simulink model "Bio_fedbatch_PP2"  (R2022a)
settings: Solver=ode15s  StartTime=0.0  StopTime=tsim  RelTol=1e-4  AbsTol=1e-4
values from neighbouring files (symbols this model uses):
  Ts = 0.1    [BiofedBatchDT.m]    (also in Executable1.m; identification.m)
undefined symbols (not defined in the file or in its folder): in
libraries: sharedTrackingLibrary x1
settings Model: SimulationMode=accelerator  Creator=DELL  LastModifiedBy=LADES
settings SolverCC: SolverResetMethod=Robust
settings DataIOCC: ReturnWorkspaceOutputs=off

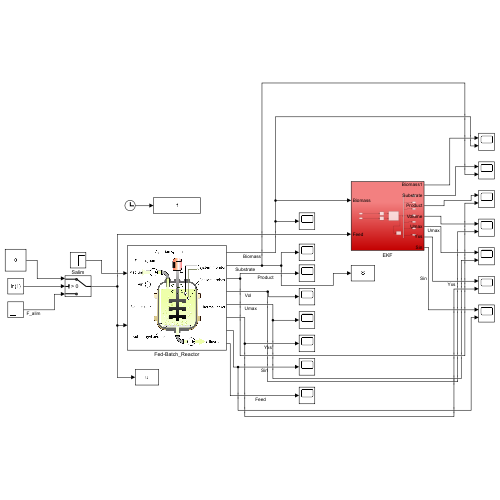
[thumbnail: Simulink's stored preview of the top-level diagram]
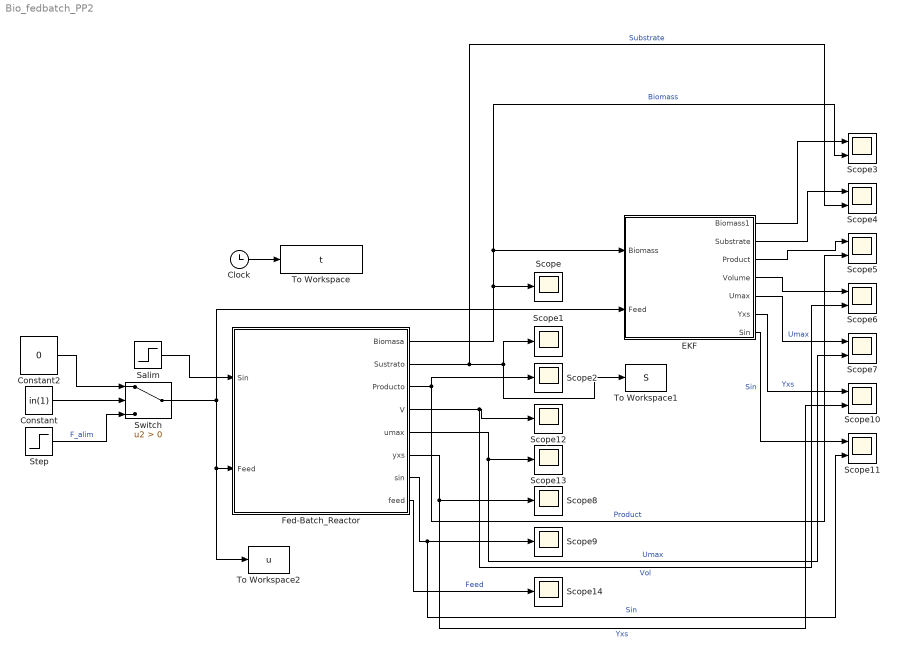
== system Bio_fedbatch_PP2 ==
  Clock : Clock
  Constant : Constant  Value=in(1)
  Constant2 : Constant  Value=0
  EKF : Subsystem
  Fed-Batch_Reactor : Subsystem
      mask Display: image('biorreactor.png'); % Use "Edit Image" on toolstrip to change.
  Salim : Step  Time=12  Before=10  After=10  SampleTime=0.1
  Scope{,1..2,8..9,12..14} (8 alike) : Scope
  Scope{3..7,10..11} (7 alike) : Scope  NumInputPorts=2
  Step : Step  Time=12  After=0.1  SampleTime=0
  Switch : Switch  Criteria=u2 > Threshold  SaturateOnIntegerOverflow=off  InputSameDT=off
  To Workspace : ToWorkspace  VariableName=t  SampleTime=0.1
  To Workspace1 : ToWorkspace  VariableName=S  SampleTime=0.1
  To Workspace2 : ToWorkspace  VariableName=u  SampleTime=0.1
  wires:
  Clock/1 -> To Workspace/1
  Fed-Batch_Reactor/2(Sustrato) -> Scope4/2, Scope1/1, To Workspace1/1  "Substrate"
  Fed-Batch_Reactor/1(Biomasa) -> EKF/1(Biomass), Scope3/2, Scope/1  "Biomass"
  Fed-Batch_Reactor/3(Producto) -> Scope2/1, Scope5/2  "Product"
  Fed-Batch_Reactor/6(yxs) -> Scope10/2, Scope8/1  "Yxs"
  Fed-Batch_Reactor/7(sin) -> Scope11/2, Scope9/1  "Sin"
  Fed-Batch_Reactor/4(V) -> Scope6/2, Scope12/1  "Vol"
  Fed-Batch_Reactor/5(umax) -> Scope7/2, Scope13/1  "Umax"
  Fed-Batch_Reactor/8(feed) -> Scope14/1  "Feed"
  Switch/1 -> To Workspace2/1, Fed-Batch_Reactor/2(Feed), EKF/2(Feed)
  EKF/1(Biomass1) -> Scope3/1
  EKF/2(Substrate) -> Scope4/1
  EKF/3(Product) -> Scope5/1
  EKF/4(Volume) -> Scope6/1
  EKF/5(Umax) -> Scope7/1  "Umax"
  EKF/6(Yxs) -> Scope10/1  "Yxs"
  EKF/7(Sin) -> Scope11/1  "Sin"
  Constant/1 -> Switch/2
  Constant2/1 -> Switch/1
  Step/1 -> Switch/3  "F_alim"
  Salim/1 -> Fed-Batch_Reactor/1(Sin)

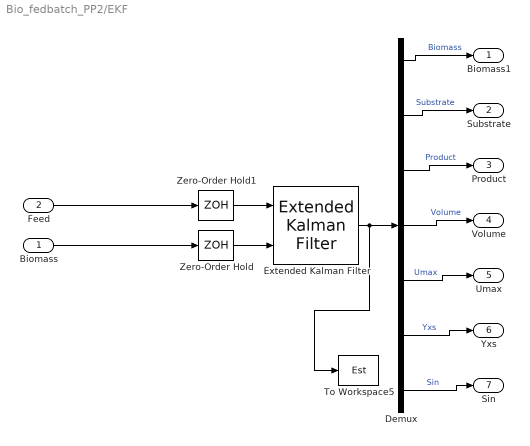
== system Bio_fedbatch_PP2/EKF ==
  Biomass : Inport
  Feed : Inport  Port=2
  Demux : Demux  Outputs=7
  Extended Kalman Filter : sharedTrackingLibrary/Extended Kalman Filter  StateTransitionFcn=BiofedBatchDT  HasStateTransitionJacobianFcn=off  HasAdditiveProcessNoise=Additive  ProcessNoise=[1e-3 1e-5 1e-3 1e-3 1e-1 1e-1 1e-1]  HasTimeVaryingProcessNoise=off  HasStateTransitionFcnExtraArgument=1  InitialState=x0  InitialStateCovariance=[1e-3 1e-5 1e-3 1e-3 1e-1 1e-1 1e-1]  MeasurementFcn1=FedBatchMeasFcn  HasMeasurementJacobianFcn1=off  HasMeasurementEnablePort1=off  HasAdditiveMeasurementNoise1=Additive  MeasurementNoise1=1e-3  HasTimeVaryingMeasurementNoise1=off  HasMeasurementFcnExtraArgument1=0  HasMeasurementWrapping1=off  MeasurementFcn2=myMeasurementFcn  HasMeasurementJacobianFcn2=off  HasMeasurementEnablePort2=off  HasAdditiveMeasurementNoise2=Additive  MeasurementNoise2=1  HasTimeVaryingMeasurementNoise2=off  HasMeasurementFcnExtraArgument2=0  HasMeasurementWrapping2=off  MeasurementFcn3=myMeasurementFcn  HasMeasurementJacobianFcn3=off  HasMeasurementEnablePort3=off  HasAdditiveMeasurementNoise3=Additive  MeasurementNoise3=1  HasTimeVaryingMeasurementNoise3=off  HasMeasurementFcnExtraArgument3=0  HasMeasurementWrapping3=off  MeasurementFcn4=myMeasurementFcn  HasMeasurementJacobianFcn4=off  HasMeasurementEnablePort4=off  HasAdditiveMeasurementNoise4=Additive  MeasurementNoise4=1  HasTimeVaryingMeasurementNoise4=off  HasMeasurementFcnExtraArgument4=0  HasMeasurementWrapping4=off  MeasurementFcn5=myMeasurementFcn  HasMeasurementJacobianFcn5=off  HasMeasurementEnablePort5=off  HasAdditiveMeasurementNoise5=Additive  MeasurementNoise5=1  HasTimeVaryingMeasurementNoise5=off  HasMeasurementFcnExtraArgument5=0  HasMeasurementWrapping5=off  EnableMultirate=off  StateTransitionFcnSampleTime=1  MeasurementFcn1SampleTime=1  MeasurementFcn2SampleTime=1  MeasurementFcn3SampleTime=1  MeasurementFcn4SampleTime=1  MeasurementFcn5SampleTime=1  UseCurrentEstimator=on  OutputStateCovariance=off  DataType=double  SampleTime=Ts  NumberOfMeasurements=1
      settings: SourceProductBaseCode=TF,AE,PW,CT,DR,ID,LP,NV,AR,RO,RR,UV,VE
  To Workspace5 : ToWorkspace  VariableName=Est  SampleTime=0.1
  Zero-Order Hold : ZeroOrderHold  SampleTime=Ts
  Zero-Order Hold1 : ZeroOrderHold  SampleTime=Ts
  Biomass1 : Outport
  Substrate : Outport  Port=2
  Product : Outport  Port=3
  Volume : Outport  Port=4
  Umax : Outport  Port=5
  Yxs : Outport  Port=6
  Sin : Outport  Port=7
  wires:
  Extended Kalman Filter/1 -> To Workspace5/1, Demux/1
  Demux/6 -> Yxs/1  "Yxs"
  Demux/2 -> Substrate/1  "Substrate"
  Feed/1 -> Zero-Order Hold1/1
  Zero-Order Hold/1 -> Extended Kalman Filter/2
  Zero-Order Hold1/1 -> Extended Kalman Filter/1
  Demux/1 -> Biomass1/1  "Biomass"
  Biomass/1 -> Zero-Order Hold/1
  Demux/4 -> Volume/1  "Volume"
  Demux/7 -> Sin/1  "Sin"
  Demux/3 -> Product/1  "Product"
  Demux/5 -> Umax/1  "Umax"

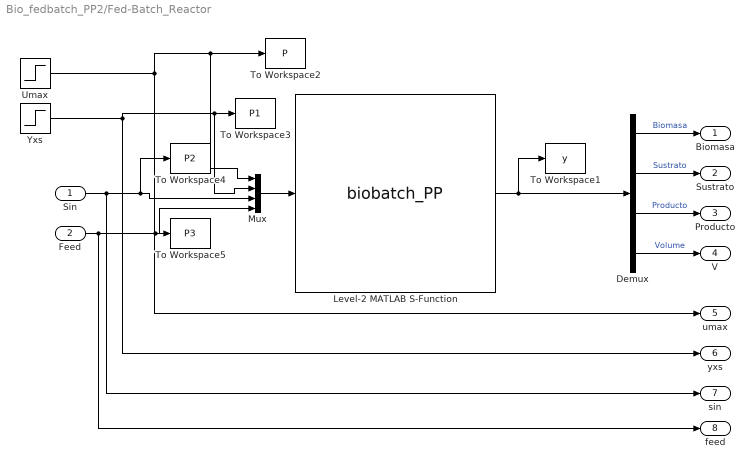
== system Bio_fedbatch_PP2/Fed-Batch_Reactor ==
  Sin : Inport
  Feed : Inport  Port=2
  Demux : Demux
  Level-2 MATLAB S-Function : M-S-Function  FunctionName=biobatch_PP  Parameters=0.01, 20, 0,1
      mask Display: image('biorreactor.png'); % Use "Edit Image" on toolstrip to change.
  Mux : Mux
  To Workspace1 : ToWorkspace  VariableName=y  SampleTime=0.1
  To Workspace2 : ToWorkspace  VariableName=P  SampleTime=0.1
  To Workspace3 : ToWorkspace  VariableName=P1  SampleTime=0.1
  To Workspace4 : ToWorkspace  VariableName=P2  SampleTime=0.1
  To Workspace5 : ToWorkspace  VariableName=P3  SampleTime=0.1
  Umax : Step  Time=0  Before=0.83  After=0.83  SampleTime=0.1
  Yxs : Step  Time=0  Before=0.8  After=0.8  SampleTime=0.1
  Biomasa : Outport
  Sustrato : Outport  Port=2
  Producto : Outport  Port=3
  V : Outport  Port=4
  umax : Outport  Port=5
  yxs : Outport  Port=6
  sin : Outport  Port=7
  feed : Outport  Port=8
  wires:
  Level-2 MATLAB S-Function/1 -> Demux/1, To Workspace1/1
  Mux/1 -> Level-2 MATLAB S-Function/1
  Yxs/1 -> Mux/2, To Workspace3/1, yxs/1
  Demux/2 -> Sustrato/1  "Sustrato"
  Umax/1 -> umax/1, Mux/1, To Workspace2/1
  Demux/3 -> Producto/1  "Producto"
  Demux/1 -> Biomasa/1  "Biomasa"
  Sin/1 -> sin/1, To Workspace4/1, Mux/3
  Feed/1 -> feed/1, Mux/4, To Workspace5/1
  Demux/4 -> V/1  "Volume"
